simulink library "Contact_Forces_Lib"  (R2018a)
settings: Solver=ode45  StartTime=0.0  StopTime=10.0  RelTol=1e-3  EnableMultiTasking=on
undefined symbols (not defined in the file or in its folder): b_contact, custom_param_1, custom_param_2, k_contact, l_cone, length_cylinder, length_tube, mu_kinetic, mu_static, pen_exponent, pen_full_damp_F, rad_s_cone, radius_cylinder, radius_tube, v_thr, X, Y, Z
libraries: nesl_utility x153, sm_lib x64, $bdroot x53, simulink x9, fl_lib x1
(part 6 of 7)

== system Contact_Forces_Lib/3D/Sphere to Tube Force/Sensing/rad_azm_cal ==
  X : Inport
  Y : Inport  Port=2
  Xdot : Inport  Port=3
  Ydot : Inport  Port=4
  Demux : Demux
  If centers are not colocated : If  IfExpression=(u1 > 0)
  Math Function : Math  Operator=square  SaturateOnIntegerOverflow=on
  Math Function1 : Math  Operator=square  SaturateOnIntegerOverflow=on
  Merge : Merge  InitialOutput=0  InputPortOffsets=0
  Sum : Sum  Inputs=|++
  rad_0 : Subsystem
  rad_azm_cal : Subsystem
  rad : Outport
  azm : Outport  Port=2
  radv : Outport  Port=3
  azmv : Outport  Port=4
  wires:
  Merge/1 -> Demux/1
  If centers are not colocated/1 -> rad_azm_cal/Action
  If centers are not colocated/2 -> rad_0/Action
  Demux/2 -> azm/1
  rad_0/1(F) -> Merge/1
  Demux/4 -> azmv/1
  Demux/1 -> rad/1
  Demux/3 -> radv/1
  Xdot/1 -> rad_azm_cal/3(Xdot)
  X/1 -> Math Function/1, rad_azm_cal/1(X)
  Ydot/1 -> rad_azm_cal/4(Ydot)
  Y/1 -> Math Function1/1, rad_azm_cal/2(Y)
  rad_azm_cal/1(F) -> Merge/2
  Math Function1/1 -> Sum/2
  Math Function/1 -> Sum/1
  Sum/1 -> If centers are not colocated/1

== system Contact_Forces_Lib/Friction Utilities/Utilities/Product/FcConst ==
  PS Product : fl_lib/Physical Signals/Functions/PS Product
      settings: SourceProductName=Simscape
  PS-Simulink Converter2 : nesl_utility/PS-Simulink Converter  PhysicalDomain=network_engine_domain  SubClassName=ps_output  LeftPortType=input  RightPortType=output  PseudoPeriodic=off  Frequencies=[]  Unit=1  AffineConversion=off
  Terminator : Terminator
  Fc : PMIOPort  Side=Right
  v : PMIOPort  Port=2  Side=Right
  wires:
  PS-Simulink Converter2/1 -> Terminator/1
  connections:
  PS Product/LConn1 -- v/RConn1
  PS Product/LConn2 -- Fc/RConn1
  PS-Simulink Converter2/LConn1 -- PS Product/RConn1

== system Contact_Forces_Lib/Friction Utilities/Utilities/Product/FcVect ==
  PS-Simulink Converter1 : nesl_utility/PS-Simulink Converter  PhysicalDomain=network_engine_domain  SubClassName=ps_output  LeftPortType=input  RightPortType=output  PseudoPeriodic=off  Frequencies=[]  Unit=1  AffineConversion=off
  PS-Simulink Converter2 : nesl_utility/PS-Simulink Converter  PhysicalDomain=network_engine_domain  SubClassName=ps_output  LeftPortType=input  RightPortType=output  PseudoPeriodic=off  Frequencies=[]  Unit=1  AffineConversion=off
  Terminator : Terminator
  Terminator1 : Terminator
  Fc : PMIOPort  Side=Right
  v : PMIOPort  Port=2  Side=Right
  wires:
  PS-Simulink Converter1/1 -> Terminator1/1
  PS-Simulink Converter2/1 -> Terminator/1
  connections:
  PS-Simulink Converter1/LConn1 -- Fc/RConn1
  PS-Simulink Converter2/LConn1 -- v/RConn1

== system Contact_Forces_Lib/2D/Circle to Circle Force/Ff/Resolve Ff/Ff in CirB ==
  Ff : Inport
  azm : Inport  Port=2
  Divide1 : Product  Inputs=**
  Divide2 : Product  Inputs=**
  Gain3 : Gain  Gain=-1
  cos : Trigonometry
  deg2rad : Gain  Gain=pi/180
  sin : Trigonometry  Operator=cos
  FxCirB : Outport
  FyCirB : Outport  Port=2
  wires:
  Gain3/1 -> Divide1/2
  Ff/1 -> Divide1/1, Divide2/1
  Divide1/1 -> FxCirB/1
  deg2rad/1 -> cos/1, sin/1
  sin/1 -> Divide2/2
  cos/1 -> Gain3/1
  Divide2/1 -> FyCirB/1  "Fy Cir"
  azm/1 -> deg2rad/1

== system Contact_Forces_Lib/2D/Circle to Circle Force/Ff/Resolve Ff/Ff in CirF ==
  R : Inport
  FxCirB : Inport  Port=2
  FyCirB : Inport  Port=3
  Demux : Demux  Outputs=2
  Divide3 : Product  Inputs=**  Multiplication=Matrix(*)
  Gain1 : Gain  Gain=-1
  Mux1 : Mux  Inputs=2
  FyCirF : Outport
  FxCirF : Outport  Port=2
  wires:
  FxCirB/1 -> Mux1/2
  FyCirB/1 -> Mux1/1
  Demux/2 -> FxCirF/1
  Demux/1 -> FyCirF/1
  Gain1/1 -> Demux/1
  Mux1/1 -> Divide3/2
  Divide3/1 -> Gain1/1
  R/1 -> Divide3/1

== system Contact_Forces_Lib/2D/Circle to Circle Force/Ff/Resolve Ff/Tz ==
  Ff : Inport
  Base Radius : Constant  Value=cirB_rad
  Divide4 : Product  Inputs=**
  Divide5 : Product  Inputs=**
  Follower Radius : Constant  Value=cirF_rad
  Gain2 : Gain
  TzB : Outport
  TzF : Outport  Port=2
  wires:
  Ff/1 -> Divide4/2, Gain2/1
  Gain2/1 -> Divide5/1
  Divide4/1 -> TzF/1
  Follower Radius/1 -> Divide4/1
  Divide5/1 -> TzB/1
  Base Radius/1 -> Divide5/2

== system Contact_Forces_Lib/2D/Circle to Circle Force Enabled/Ff/Resolve Ff/Ff in CirB ==
  Ff : Inport
  azm : Inport  Port=2
  Divide1 : Product  Inputs=**
  Divide2 : Product  Inputs=**
  Gain3 : Gain  Gain=-1
  cos : Trigonometry
  deg2rad : Gain  Gain=pi/180
  sin : Trigonometry  Operator=cos
  FxCirB : Outport
  FyCirB : Outport  Port=2
  wires:
  azm/1 -> deg2rad/1
  Divide2/1 -> FyCirB/1  "Fy Cir"
  cos/1 -> Gain3/1
  sin/1 -> Divide2/2
  deg2rad/1 -> sin/1, cos/1
  Divide1/1 -> FxCirB/1
  Ff/1 -> Divide2/1, Divide1/1
  Gain3/1 -> Divide1/2

== system Contact_Forces_Lib/2D/Circle to Circle Force Enabled/Ff/Resolve Ff/Ff in CirF ==
  R : Inport
  FxCirB : Inport  Port=2
  FyCirB : Inport  Port=3
  Demux : Demux  Outputs=2
  Divide3 : Product  Inputs=**  Multiplication=Matrix(*)
  Gain1 : Gain  Gain=-1
  Mux1 : Mux  Inputs=2
  FyCirF : Outport
  FxCirF : Outport  Port=2
  wires:
  R/1 -> Divide3/1
  Divide3/1 -> Gain1/1
  Mux1/1 -> Divide3/2
  Gain1/1 -> Demux/1
  Demux/1 -> FyCirF/1
  Demux/2 -> FxCirF/1
  FyCirB/1 -> Mux1/1
  FxCirB/1 -> Mux1/2

== system Contact_Forces_Lib/2D/Circle to Circle Force Enabled/Ff/Resolve Ff/Tz ==
  Ff : Inport
  Base Radius : Constant  Value=cirB_rad
  Divide4 : Product  Inputs=**
  Divide5 : Product  Inputs=**
  Follower Radius : Constant  Value=cirF_rad
  Gain2 : Gain
  TzB : Outport
  TzF : Outport  Port=2
  wires:
  Base Radius/1 -> Divide5/2
  Divide5/1 -> TzB/1
  Follower Radius/1 -> Divide4/1
  Divide4/1 -> TzF/1
  Gain2/1 -> Divide5/1
  Ff/1 -> Gain2/1, Divide4/2

== system Contact_Forces_Lib/2D/Circle to Finite Line Force/Forces/Resolve Forces/FnCir ==
  note: Calculate circle Normal Force in circle reference frame
  Unit Vector : Inport
  Fn : Inport  Port=2
  Demux1 : Demux  Outputs=2
  Divide1 : Product  Inputs=**
  FxCir : Outport
  FyCir : Outport  Port=2
  wires:
  Unit Vector/1 -> Divide1/2
  Divide1/1 -> Demux1/1
  Fn/1 -> Divide1/1
  Demux1/2 -> FyCir/1  "Fy Cir"
  Demux1/1 -> FxCir/1  "Fx Cir"

== system Contact_Forces_Lib/2D/Circle to Finite Line Force/Forces/Resolve Forces/FnLin ==
  note: Normal Force is calculated in line reference frame,
      | and acts along x-axis only.
  Fn : Inport
  Constant : Constant  Value=0
  Constant1 : Constant  Value=0
  Sum : Sum
  FxLin : Outport
  FyLin : Outport  Port=2
  wires:
  Constant1/1 -> Sum/1
  Sum/1 -> FxLin/1
  Fn/1 -> Sum/2  "Fx Lin"
  Constant/1 -> FyLin/1  "Fy Lin"

== system Contact_Forces_Lib/2D/Circle to Finite Line Force/Forces/Resolve Forces/Friction ==
  Unit Vector : Inport
  Fn : Inport  Port=2
  X Sep : Inport  Port=3
  vLin : Inport  Port=4
  wz : Inport  Port=5
  Components : Gain  Gain=[1 -1]
  Demux : Demux  Outputs=2
  Friction Law : $bdroot/Friction Law  OverrideUsingVariant=None
  Line Ref h : Gain  Gain=line_depth
  Product1 : Product
  Product2 : Product
  Product3 : Product
  Radius : Gain  Gain=-circle_rad
  Sign : Signum
  Sum : Sum  Inputs=-+
  VCirPt : Subsystem
  FxCir : Outport
  FyCir : Outport  Port=2
  FyLin : Outport  Port=3
  TzLin : Outport  Port=4
  TzCir : Outport  Port=5
  Ff : Outport  Port=6
  wires:
  Sign/1 -> Product3/2, Product1/2
  X Sep/1 -> VCirPt/2(X sep), Sign/1
  Product2/1 -> Demux/1
  Radius/1 -> TzCir/1
  Line Ref h/1 -> TzLin/1
  Fn/1 -> Friction Law/1
  Sum/1 -> Friction Law/2
  Unit Vector/1 -> Components/1
  wz/1 -> VCirPt/1(wz)
  Demux/2 -> FxCir/1  "FxCir"
  VCirPt/1(vCir) -> Sum/2
  vLin/1 -> Sum/1
  Demux/1 -> FyCir/1  "FyCir"
  Friction Law/1 -> Product1/1, Radius/1, Ff/1, Product2/2, Line Ref h/1  "Ff"
  Product1/1 -> FyLin/1
  Components/1 -> Product3/1
  Product3/1 -> Product2/1

== system Contact_Forces_Lib/2D/Circle to Finite Line Force Enabled/Forces/Resolve Forces/FnCir ==
  note: Calculate circle Normal Force in circle reference frame
  Unit Vector : Inport
  Fn : Inport  Port=2
  Demux1 : Demux  Outputs=2
  Divide1 : Product  Inputs=**
  FxCir : Outport
  FyCir : Outport  Port=2
  wires:
  Demux1/1 -> FxCir/1  "Fx Cir"
  Demux1/2 -> FyCir/1  "Fy Cir"
  Fn/1 -> Divide1/1
  Divide1/1 -> Demux1/1
  Unit Vector/1 -> Divide1/2

== system Contact_Forces_Lib/2D/Circle to Finite Line Force Enabled/Forces/Resolve Forces/FnLin ==
  note: Normal Force is calculated in line reference frame,
      | and acts along x-axis only.
  Fn : Inport
  Constant : Constant  Value=0
  Constant1 : Constant  Value=0
  Sum : Sum
  FxLin : Outport
  FyLin : Outport  Port=2
  wires:
  Constant/1 -> FyLin/1  "Fy Lin"
  Fn/1 -> Sum/2  "Fx Lin"
  Sum/1 -> FxLin/1
  Constant1/1 -> Sum/1

== system Contact_Forces_Lib/2D/Circle to Finite Line Force Enabled/Forces/Resolve Forces/Friction ==
  Unit Vector : Inport
  Fn : Inport  Port=2
  X Sep : Inport  Port=3
  vLin : Inport  Port=4
  wz : Inport  Port=5
  Components : Gain  Gain=[1 -1]
  Demux : Demux  Outputs=2
  Friction Law : $bdroot/Friction Law  OverrideUsingVariant=None
  Line Ref h : Gain  Gain=line_depth
  Product1 : Product
  Product2 : Product
  Product3 : Product
  Radius : Gain  Gain=-circle_rad
  Sign : Signum
  Sum : Sum  Inputs=-+
  VCirPt : Subsystem
  FxCir : Outport
  FyCir : Outport  Port=2
  FyLin : Outport  Port=3
  TzLin : Outport  Port=4
  TzCir : Outport  Port=5
  Ff : Outport  Port=6
  wires:
  Product3/1 -> Product2/1
  Components/1 -> Product3/1
  Product1/1 -> FyLin/1
  Friction Law/1 -> Line Ref h/1, Product2/2, Ff/1, Radius/1, Product1/1  "Ff"
  Demux/1 -> FyCir/1  "FyCir"
  vLin/1 -> Sum/1
  VCirPt/1(vCir) -> Sum/2
  Demux/2 -> FxCir/1  "FxCir"
  wz/1 -> VCirPt/1(wz)
  Unit Vector/1 -> Components/1
  Sum/1 -> Friction Law/2
  Fn/1 -> Friction Law/1
  Line Ref h/1 -> TzLin/1
  Radius/1 -> TzCir/1
  Product2/1 -> Demux/1
  X Sep/1 -> Sign/1, VCirPt/2(X sep)
  Sign/1 -> Product1/2, Product3/2

== system Contact_Forces_Lib/2D/Circle to Ring Force/Forces/Ff/Resolve Ff ==
  note: Resolve Friction Force in
      | Circle B reference frame
      | Sign of Fn indicates
      | inside or outside ring.
  note: Resolve Friction Force in
      | Circle F reference frame
  Fn : Inport
  R : Inport  Port=2
  Ff : Inport  Port=3
  azm : Inport  Port=4
  Ff in CirB : Subsystem
  Ff in CirF : Subsystem
  Product : Product
  Sign : Signum  ZeroCross=off
  Tz : Subsystem
  FxCirF : Outport
  FyCirF : Outport  Port=2
  TzCirF : Outport  Port=3
  FxRinB : Outport  Port=4
  FyRinB : Outport  Port=5
  TzRinB : Outport  Port=6
  wires:
  Product/1 -> Ff in CirB/1(Ff)
  Sign/1 -> Product/2
  Fn/1 -> Sign/1
  Ff in CirF/1(FyCirF) -> FyCirF/1
  Ff in CirB/1(FxRinB) -> FxRinB/1, Ff in CirF/2(FxRinB)
  Ff in CirB/2(FyRinB) -> FyRinB/1, Ff in CirF/3(FyRinB)
  Ff in CirF/2(FxCirF) -> FxCirF/1
  Ff/1 -> Product/1, Tz/1(Ff)
  Tz/1(TzRinB) -> TzRinB/1
  Tz/2(TzCirF) -> TzCirF/1
  azm/1 -> Ff in CirB/2(azm)
  R/1 -> Ff in CirF/1(R)

== system Contact_Forces_Lib/2D/Circle to Ring Force/Forces/Ff/vTan ==
  Fn : Inport
  rad : Inport  Port=2
  Pen : Inport  Port=3
  vazm : Inport  Port=4
  wzf : Inport  Port=5
  Follower Radius : Constant  Value=radius_circle
  Midpt Pen : Gain  Gain=0.5
  Product1 : Product
  Product2 : Product
  Product3 : Product  Inputs=3
  Sign : Signum  ZeroCross=off
  Sum : Sum  Inputs=++-
  Sum1 : Sum  Inputs=+-
  Sum2 : Sum  Inputs=-+
  vTan : Outport
  wires:
  Sign/1 -> Product1/2, Product3/3
  Fn/1 -> Sign/1
  Product1/1 -> Sum/3
  Sum2/1 -> vTan/1
  Pen/1 -> Midpt Pen/1
  Sum/1 -> Product2/2
  rad/1 -> Sum/2
  Product2/1 -> Sum2/2  "vTan in B"
  Product3/1 -> Sum2/1  "vTan of F"
  Follower Radius/1 -> Sum1/1, Product1/1
  wzf/1 -> Product3/1
  vazm/1 -> Product2/1
  Midpt Pen/1 -> Sum1/2, Sum/1
  Sum1/1 -> Product3/2

== system Contact_Forces_Lib/2D/Circle to Ring Force/Forces/Fn/Fn in CirB ==
  Fn : Inport
  azm : Inport  Port=2
  Divide1 : Product  Inputs=**
  Divide2 : Product  Inputs=**
  Gain2 : Gain  Gain=-1
  cos : Trigonometry  Operator=cos
  deg2rad : Gain  Gain=pi/180
  sin : Trigonometry
  FxCirB : Outport
  FyCirB : Outport  Port=2
  wires:
  Gain2/1 -> Divide1/1, Divide2/1
  deg2rad/1 -> cos/1, sin/1
  sin/1 -> Divide2/2
  cos/1 -> Divide1/2
  Divide1/1 -> FxCirB/1
  Divide2/1 -> FyCirB/1
  Fn/1 -> Gain2/1
  azm/1 -> deg2rad/1

== system Contact_Forces_Lib/2D/Circle to Ring Force/Forces/Fn/Fn in CirF ==
  R : Inport
  FxCirB : Inport  Port=2
  FyCirB : Inport  Port=3
  Demux : Demux  Outputs=2
  Divide3 : Product  Inputs=**  Multiplication=Matrix(*)
  Gain : Gain  Gain=-1
  Mux1 : Mux  Inputs=2
  FyCirF : Outport
  FxCirF : Outport  Port=2
  wires:
  Demux/2 -> FxCirF/1
  Demux/1 -> FyCirF/1
  Gain/1 -> Demux/1
  Mux1/1 -> Divide3/2
  Divide3/1 -> Gain/1
  R/1 -> Divide3/1
  FyCirB/1 -> Mux1/1
  FxCirB/1 -> Mux1/2

== system Contact_Forces_Lib/2D/Composite Forces/Box to Belt Force/Belt Ends/Sensing C5 ==
  S : Inport
  Bus Selector : BusSelector  OutputSignals=Normal Force
  Fn : Outport
  wires:
  S/1 -> Bus Selector/1
  Bus Selector/1 -> Fn/1  "<Normal Force>"

== system Contact_Forces_Lib/2D/Composite Forces/Box to Belt Force/Belt Ends/Sensing C6 ==
  S : Inport
  Bus Selector : BusSelector  OutputSignals=Normal Force
  Fn : Outport
  wires:
  Bus Selector/1 -> Fn/1  "<Normal Force>"
  S/1 -> Bus Selector/1

== system Contact_Forces_Lib/2D/Composite Forces/Box to Belt Force/Belt Ends/Sensing C7 ==
  S : Inport
  Bus Selector : BusSelector  OutputSignals=Normal Force
  Fn : Outport
  wires:
  Bus Selector/1 -> Fn/1  "<Normal Force>"
  S/1 -> Bus Selector/1

== system Contact_Forces_Lib/2D/Composite Forces/Box to Belt Force/Belt Ends/Sensing C8 ==
  S : Inport
  Bus Selector : BusSelector  OutputSignals=Normal Force
  Fn : Outport
  wires:
  S/1 -> Bus Selector/1
  Bus Selector/1 -> Fn/1  "<Normal Force>"

== system Contact_Forces_Lib/2D/Composite Forces/Box to Belt Force/Belt Faces/Sensing C1 ==
  S : Inport
  Bus Selector : BusSelector  OutputSignals=Normal Force
  Fn : Outport
  wires:
  Bus Selector/1 -> Fn/1  "<Normal Force>"
  S/1 -> Bus Selector/1

== system Contact_Forces_Lib/2D/Composite Forces/Box to Belt Force/Belt Faces/Sensing C2 ==
  S : Inport
  Bus Selector : BusSelector  OutputSignals=Normal Force
  Fn : Outport
  wires:
  S/1 -> Bus Selector/1
  Bus Selector/1 -> Fn/1  "<Normal Force>"

== system Contact_Forces_Lib/2D/Composite Forces/Box to Belt Force/Belt Faces/Sensing C3 ==
  S : Inport
  Bus Selector : BusSelector  OutputSignals=Normal Force
  Fn : Outport
  wires:
  S/1 -> Bus Selector/1
  Bus Selector/1 -> Fn/1  "<Normal Force>"

== system Contact_Forces_Lib/2D/Composite Forces/Box to Belt Force/Belt Faces/Sensing C4 ==
  S : Inport
  Bus Selector : BusSelector  OutputSignals=Normal Force
  Fn : Outport
  wires:
  Bus Selector/1 -> Fn/1  "<Normal Force>"
  S/1 -> Bus Selector/1

== system Contact_Forces_Lib/2D/Composite Forces/Box to Box Force/BoxB Corners/Forces ==
  1AC : Inport
  1BD : Inport  Port=2
  2AC : Inport  Port=3
  2BD : Inport  Port=4
  3AC : Inport  Port=5
  3BD : Inport  Port=6
  4AC : Inport  Port=7
  4BD : Inport  Port=8
  Bus Creator : BusCreator  Inputs=8
  Bus Selector{1..8} (8 alike) : BusSelector  OutputSignals=FLin.Fx  OutputAsBus=on
  tag scope: FrcBC=scoped
  wires:
  Bus Creator/1 -> [FrcBC]
  Bus Selector7/1 -> Bus Creator/8  "BC4BD"
  4BD/1 -> Bus Selector7/1
  Bus Selector8/1 -> Bus Creator/7  "BC4AC"
  4AC/1 -> Bus Selector8/1
  Bus Selector5/1 -> Bus Creator/6  "BC3BD"
  3BD/1 -> Bus Selector5/1
  Bus Selector6/1 -> Bus Creator/5  "BC3AC"
  3AC/1 -> Bus Selector6/1
  Bus Selector3/1 -> Bus Creator/4  "BC2BD"
  2BD/1 -> Bus Selector3/1
  Bus Selector4/1 -> Bus Creator/3  "BC2AC"
  2AC/1 -> Bus Selector4/1
  Bus Selector1/1 -> Bus Creator/2  "BC1BD"
  1BD/1 -> Bus Selector1/1
  Bus Selector2/1 -> Bus Creator/1  "BC1AC"
  1AC/1 -> Bus Selector2/1

== system Contact_Forces_Lib/2D/Composite Forces/Box to Box Force/BoxF Corners/Forces ==
  1AC : Inport
  1BD : Inport  Port=2
  2AC : Inport  Port=3
  2BD : Inport  Port=4
  3AC : Inport  Port=5
  3BD : Inport  Port=6
  4AC : Inport  Port=7
  4BD : Inport  Port=8
  Bus Creator : BusCreator  Inputs=8
  Bus Selector{1..8} (8 alike) : BusSelector  OutputSignals=FLin.Fx  OutputAsBus=on
  tag scope: FrcFC=scoped
  wires:
  Bus Creator/1 -> [FrcFC]
  Bus Selector7/1 -> Bus Creator/8  "FC4BD"
  4BD/1 -> Bus Selector7/1
  Bus Selector8/1 -> Bus Creator/7  "FC4AC"
  4AC/1 -> Bus Selector8/1
  Bus Selector5/1 -> Bus Creator/6  "FC3BD"
  3BD/1 -> Bus Selector5/1
  Bus Selector6/1 -> Bus Creator/5  "FC3AC"
  3AC/1 -> Bus Selector6/1
  Bus Selector3/1 -> Bus Creator/4  "FC2BD"
  2BD/1 -> Bus Selector3/1
  Bus Selector4/1 -> Bus Creator/3  "FC2AC"
  2AC/1 -> Bus Selector4/1
  Bus Selector1/1 -> Bus Creator/2  "FC1BD"
  1BD/1 -> Bus Selector1/1
  Bus Selector2/1 -> Bus Creator/1  "FC1AC"
  1AC/1 -> Bus Selector2/1

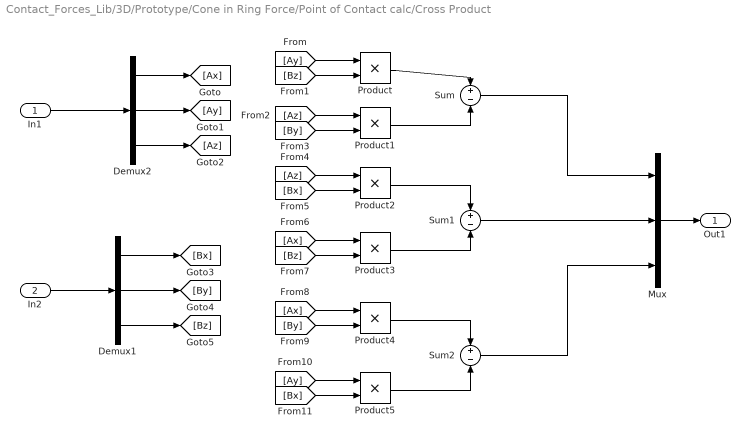
== system Contact_Forces_Lib/3D/Prototype/Cone in Ring Force/Point of Contact calc/Cross Product ==
  In1 : Inport
  In2 : Inport  Port=2
  Demux1 : Demux  Outputs=3
  Demux2 : Demux  Outputs=3
  Mux : Mux  Inputs=3
  Product{,1..5} (6 alike) : Product
  Sum : Sum  Inputs=+|-
  Sum1 : Sum  Inputs=+|-
  Sum2 : Sum  Inputs=+|-
  Out1 : Outport
  wires:
  [Bx] -> Product5/2
  [Ay] -> Product5/1
  [By] -> Product4/2
  [Ax] -> Product4/1
  [Bz] -> Product3/2
  [Ax] -> Product3/1
  [Bx] -> Product2/2
  [Az] -> Product2/1
  [By] -> Product1/2
  [Az] -> Product1/1
  [Bz] -> Product/2
  [Ay] -> Product/1
  Demux1/3 -> [Bz]
  Demux1/2 -> [By]
  Demux1/1 -> [Bx]
  Demux2/3 -> [Az]
  Demux2/2 -> [Ay]
  Demux2/1 -> [Ax]
  In1/1 -> Demux2/1
  Sum2/1 -> Mux/3
  Sum/1 -> Mux/1
  Sum1/1 -> Mux/2
  Product5/1 -> Sum2/2
  Product4/1 -> Sum2/1
  Product3/1 -> Sum1/2
  Product2/1 -> Sum1/1
  Product/1 -> Sum/1
  Product1/1 -> Sum/2
  Mux/1 -> Out1/1
  In2/1 -> Demux1/1

== system Contact_Forces_Lib/3D/Prototype/Cone in Ring Force/Point of Contact calc/Force Calc ==
  x : Inport
  y : Inport  Port=2
  r : Inport  Port=3
  z : Inport  Port=4
  th : Inport  Port=5
  Computing Force from nonzero penetration points : Subsystem  Commented=on
  Constant2 : Constant  Value=r_tube
  Dead Zone : DeadZone  LowerValue=-inf  UpperValue=0  ZeroCross=off  SaturateOnIntegerOverflow=on
  MAX_ML : Subsystem  Commented=on
  MAX_SL : Subsystem
  Math Function : Math  Operator=square  SaturateOnIntegerOverflow=on
  Math Function1 : Math  Operator=square  SaturateOnIntegerOverflow=on
  Reciprocal Sqrt : Sqrt  SaturateOnIntegerOverflow=on
  Sum : Sum  Inputs=|++
  Sum1 : Sum  Inputs=|+-
  Fx : Outport
  Fy : Outport  Port=2
  Fz : Outport  Port=3
  pc : Outport  Port=4
  wires:
  x/1 -> MAX_SL/2(X), Math Function/1
  Sum/1 -> Reciprocal Sqrt/1
  Reciprocal Sqrt/1 -> Sum1/1
  Constant2/1 -> Sum1/2
  Sum1/1 -> Dead Zone/1
  Math Function1/1 -> Sum/1
  Math Function/1 -> Sum/2
  y/1 -> Math Function1/1, MAX_SL/1(Y)
  MAX_SL/1(Fx) -> Fx/1
  MAX_SL/2(Fy) -> Fy/1
  Dead Zone/1 -> MAX_SL/3(Pen)
  MAX_SL/3(Fz) -> Fz/1
  MAX_SL/4(pc) -> pc/1
  r/1 -> MAX_SL/4(r)
  th/1 -> MAX_SL/5(th)
  z/1 -> MAX_SL/6(z)

== system Contact_Forces_Lib/3D/Prototype/Cone in Ring Force/Point of Contact calc/r calc ==
  note: r(z) = (z+l_cyl/2)(rl-rs)/lc +rl
  z : Inport
  Constant4 : Constant  Value=(rl + (l_cyl*(rl - rs))/(2*lc))
  Gain1 : Gain  Gain=(rl - rs)/lc
  Sum1 : Sum  Inputs=|++
  r : Outport
  wires:
  Constant4/1 -> Sum1/2
  Gain1/1 -> Sum1/1
  z/1 -> Gain1/1
  Sum1/1 -> r/1

== system Contact_Forces_Lib/3D/Prototype/Cone in Ring Force/Point of Contact calc/x calc ==
  r11 : Inport
  r12 : Inport  Port=2
  r13 : Inport  Port=3
  xc : Inport  Port=4
  th : Inport  Port=5
  z : Inport  Port=6
  r : Inport  Port=7
  Product{,1..4} (5 alike) : Product
  Sum : Sum  Inputs=|++++
  Trigonometric Function : Trigonometry  Operator=cos
  Trigonometric Function1 : Trigonometry
  x : Outport
  wires:
  th/1 -> Trigonometric Function1/1, Trigonometric Function/1
  Sum/1 -> x/1
  Product/1 -> Product3/1
  Product4/1 -> Sum/3
  Trigonometric Function/1 -> Product/2
  Trigonometric Function1/1 -> Product1/2
  Product3/1 -> Sum/2
  Product1/1 -> Product4/2
  r11/1 -> Product/1
  r12/1 -> Product1/1
  xc/1 -> Sum/1
  r13/1 -> Product2/1
  z/1 -> Product2/2
  Product2/1 -> Sum/4
  r/1 -> Product3/2, Product4/1

== system Contact_Forces_Lib/3D/Prototype/Cone in Ring Force/Point of Contact calc/y calc ==
  r21 : Inport
  r22 : Inport  Port=2
  r23 : Inport  Port=3
  yc : Inport  Port=4
  th : Inport  Port=5
  z : Inport  Port=6
  r : Inport  Port=7
  Product{,1..4} (5 alike) : Product
  Sum : Sum  Inputs=|++++
  Trigonometric Function : Trigonometry  Operator=cos
  Trigonometric Function1 : Trigonometry
  y : Outport
  wires:
  Product2/1 -> Sum/4
  z/1 -> Product2/2
  r23/1 -> Product2/1
  yc/1 -> Sum/1
  r22/1 -> Product1/1
  r21/1 -> Product/1
  Product1/1 -> Product4/2
  Product3/1 -> Sum/2
  Trigonometric Function1/1 -> Product1/2
  Trigonometric Function/1 -> Product/2
  Product4/1 -> Sum/3
  Product/1 -> Product3/1
  Sum/1 -> y/1
  th/1 -> Trigonometric Function1/1, Trigonometric Function/1
  r/1 -> Product3/2, Product4/1

== system Contact_Forces_Lib/3D/Prototype/Cone in Ring Force/Point of Contact calc/z calc ==
  note: num = -(Zc - L/2 + r31*cos(th)*(rl + (Lcyl*(rl - rs))/(2*lc)) + r32*sin(th)*(rl + (Lcyl*(rl - rs))/(2*lc)))
      | den = (r33 + (r31*cos(th)*(rl - rs))/lc + (r32*sin(th)*(rl - rs))/lc)
  r31 : Inport
  r32 : Inport  Port=2
  r33 : Inport  Port=3
  zc : Inport  Port=4
  th : Inport  Port=5
  Constant : Constant  Value=(rl + (l_cyl*(rl - rs))/(2*lc))
  Constant1 : Constant  Value=l_tube/2
  Constant2 : Constant  Value=(rl - rs)/lc
  Divide : Product  Inputs=*/
  Gain : Gain  Gain=-1
  Product{,1..5} (6 alike) : Product
  Sum : Sum  Inputs=+-++
  Sum1 : Sum  Inputs=+++
  Trigonometric Function : Trigonometry  Operator=cos
  Trigonometric Function1 : Trigonometry
  z : Outport
  wires:
  Divide/1 -> z/1
  th/1 -> Trigonometric Function1/1, Trigonometric Function/1
  Trigonometric Function/1 -> Product/2
  r31/1 -> Product/1
  Trigonometric Function1/1 -> Product1/2
  r32/1 -> Product1/1
  zc/1 -> Sum/1
  Constant1/1 -> Sum/2
  Product2/1 -> Sum/3
  Product3/1 -> Sum/4
  Product/1 -> Product4/1, Product2/1
  Product1/1 -> Product3/1, Product5/1
  Constant/1 -> Product3/2, Product2/2
  Sum/1 -> Gain/1
  Product5/1 -> Sum1/3
  Product4/1 -> Sum1/2
  r33/1 -> Sum1/1
  Constant2/1 -> Product4/2, Product5/2
  Sum1/1 -> Divide/2
  Gain/1 -> Divide/1

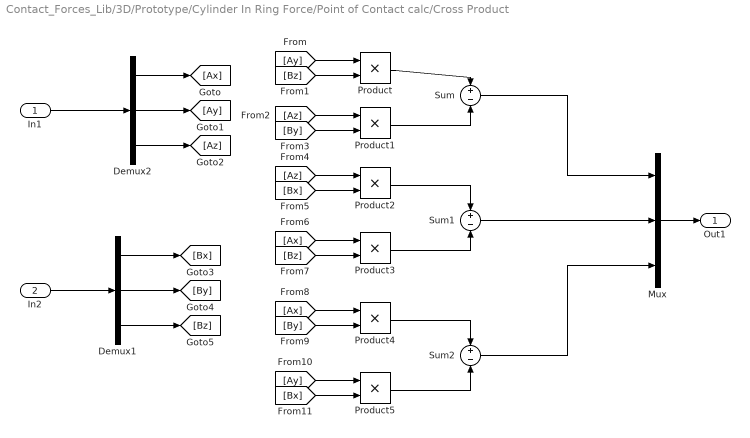
== system Contact_Forces_Lib/3D/Prototype/Cylinder In Ring Force/Point of Contact calc/Cross Product ==
  In1 : Inport
  In2 : Inport  Port=2
  Demux1 : Demux  Outputs=3
  Demux2 : Demux  Outputs=3
  Mux : Mux  Inputs=3
  Product{,1..5} (6 alike) : Product
  Sum : Sum  Inputs=+|-
  Sum1 : Sum  Inputs=+|-
  Sum2 : Sum  Inputs=+|-
  Out1 : Outport
  wires:
  [Bx] -> Product5/2
  [Ay] -> Product5/1
  [By] -> Product4/2
  [Ax] -> Product4/1
  [Bz] -> Product3/2
  [Ax] -> Product3/1
  [Bx] -> Product2/2
  [Az] -> Product2/1
  [By] -> Product1/2
  [Az] -> Product1/1
  [Bz] -> Product/2
  [Ay] -> Product/1
  Demux1/3 -> [Bz]
  Demux1/2 -> [By]
  Demux1/1 -> [Bx]
  Demux2/3 -> [Az]
  Demux2/2 -> [Ay]
  Demux2/1 -> [Ax]
  In1/1 -> Demux2/1
  Sum2/1 -> Mux/3
  Sum/1 -> Mux/1
  Sum1/1 -> Mux/2
  Product5/1 -> Sum2/2
  Product4/1 -> Sum2/1
  Product3/1 -> Sum1/2
  Product2/1 -> Sum1/1
  Product/1 -> Sum/1
  Product1/1 -> Sum/2
  Mux/1 -> Out1/1
  In2/1 -> Demux1/1

== system Contact_Forces_Lib/3D/Prototype/Cylinder In Ring Force/Point of Contact calc/Force Calc ==
  x : Inport
  y : Inport  Port=2
  v : Inport  Port=3
  z : Inport  Port=4
  th : Inport  Port=5
  Computing Force from nonzero penetration points : Subsystem  Commented=on
  Constant2 : Constant  Value=r_tube
  Dead Zone : DeadZone  LowerValue=-inf  UpperValue=0  ZeroCross=off  SaturateOnIntegerOverflow=on
  MAX_ML : Subsystem  Commented=on
  MAX_SL : Subsystem
  Math Function : Math  Operator=square  SaturateOnIntegerOverflow=on
  Math Function1 : Math  Operator=square  SaturateOnIntegerOverflow=on
  Reciprocal Sqrt : Sqrt  SaturateOnIntegerOverflow=on
  Sum : Sum  Inputs=|++
  Sum1 : Sum  Inputs=|+-
  Fx : Outport
  Fy : Outport  Port=2
  Fz : Outport  Port=3
  pc : Outport  Port=4
  maxpen : Outport  Port=5
  wires:
  y/1 -> MAX_SL/1(Y), Math Function1/1
  x/1 -> MAX_SL/2(X), Math Function/1
  Sum/1 -> Reciprocal Sqrt/1
  Reciprocal Sqrt/1 -> Sum1/1
  Constant2/1 -> Sum1/2
  Sum1/1 -> Dead Zone/1
  MAX_SL/1(Fx) -> Fx/1
  MAX_SL/2(Fy) -> Fy/1
  Dead Zone/1 -> MAX_SL/3(Pen)
  Math Function1/1 -> Sum/1
  Math Function/1 -> Sum/2
  v/1 -> MAX_SL/4(v)
  th/1 -> MAX_SL/5(th)
  z/1 -> MAX_SL/6(z)
  MAX_SL/4(pc) -> pc/1
  MAX_SL/3(Fz) -> Fz/1
  MAX_SL/5(maxpen) -> maxpen/1

== system Contact_Forces_Lib/3D/Prototype/Cylinder In Ring Force/Point of Contact calc/x calc ==
  note: Xb = r11*r*cos(th) + r12*r*sin(th) +r13*z + Xc;
  note: Find x coordinate in tube frame for cylinder point that is in the plane of the end of the tube
  r11 : Inport
  r12 : Inport  Port=2
  r13 : Inport  Port=3
  xc : Inport  Port=4
  th : Inport  Port=5
  z : Inport  Port=6
  Gain : Gain  Gain=r_cyl
  Gain1 : Gain  Gain=r_cyl
  Product : Product
  Product1 : Product
  Product2 : Product
  Sum : Sum  Inputs=|++++
  Trigonometric Function : Trigonometry  Operator=cos
  Trigonometric Function1 : Trigonometry
  x : Outport
  wires:
  th/1 -> Trigonometric Function/1, Trigonometric Function1/1
  Sum/1 -> x/1
  Product/1 -> Gain/1
  Gain1/1 -> Sum/3
  Trigonometric Function/1 -> Product/2
  Trigonometric Function1/1 -> Product1/2
  Gain/1 -> Sum/2
  Product1/1 -> Gain1/1
  r11/1 -> Product/1
  r12/1 -> Product1/1
  xc/1 -> Sum/1
  r13/1 -> Product2/1
  z/1 -> Product2/2
  Product2/1 -> Sum/4

== system Contact_Forces_Lib/3D/Prototype/Cylinder In Ring Force/Point of Contact calc/y calc ==
  note: Yb = r21*r*cos(th) + r22*r*sin(th) +r23*z + Yc;
  note: Find y coordinate in tube frame for cylinder point that is in the plane of the end of the tube
  r21 : Inport
  r22 : Inport  Port=2
  r23 : Inport  Port=3
  yc : Inport  Port=4
  th : Inport  Port=5
  z : Inport  Port=6
  Gain : Gain  Gain=r_cyl
  Gain1 : Gain  Gain=r_cyl
  Product : Product
  Product1 : Product
  Product2 : Product
  Sum : Sum  Inputs=|++++
  Trigonometric Function : Trigonometry  Operator=cos
  Trigonometric Function1 : Trigonometry
  y : Outport
  wires:
  Product2/1 -> Sum/4
  z/1 -> Product2/2
  r23/1 -> Product2/1
  yc/1 -> Sum/1
  r22/1 -> Product1/1
  r21/1 -> Product/1
  Product1/1 -> Gain1/1
  Gain/1 -> Sum/2
  Trigonometric Function1/1 -> Product1/2
  Trigonometric Function/1 -> Product/2
  Gain1/1 -> Sum/3
  Product/1 -> Gain/1
  Sum/1 -> y/1
  th/1 -> Trigonometric Function1/1, Trigonometric Function/1

== system Contact_Forces_Lib/3D/Prototype/Cylinder In Ring Force/Point of Contact calc/z calc ==
  note: Find z coordinate in cylinder frame for cylinder point that is in the plane of the end of the tube
  note: z = (L/2 - r31*r*cos(th) - r32*r*sin(th) - Zc)/r33;
  r31 : Inport
  r32 : Inport  Port=2
  r33 : Inport  Port=3
  zc : Inport  Port=4
  th : Inport  Port=5
  Constant : Constant  Value=l_tube/2
  Divide : Product  Inputs=*/
  Gain : Gain  Gain=r_cyl
  Gain1 : Gain  Gain=r_cyl
  Product : Product
  Product1 : Product
  Sum : Sum  Inputs=|---+
  Trigonometric Function : Trigonometry  Operator=cos
  Trigonometric Function1 : Trigonometry
  z : Outport
  wires:
  r32/1 -> Product1/1
  r31/1 -> Product/1
  Product1/1 -> Gain1/1
  Gain/1 -> Sum/2
  Trigonometric Function1/1 -> Product1/2
  Trigonometric Function/1 -> Product/2
  Gain1/1 -> Sum/3
  Product/1 -> Gain/1
  r33/1 -> Divide/2
  Constant/1 -> Sum/4
  Sum/1 -> Divide/1
  Divide/1 -> z/1
  zc/1 -> Sum/1
  th/1 -> Trigonometric Function1/1, Trigonometric Function/1

== system Contact_Forces_Lib/3D/Sphere in Sphere Force/Ff/Check w or v non zero/Else ==
  Action Port : ActionPort
  vabs_zero : Constant  Value=0  SampleTime=0
  vuvect_zero : Constant  Value=[0 0 0]  SampleTime=0
  vabs : Outport  InitialOutput=0
  vuvect : Outport  Port=2  InitialOutput=0
  wires:
  vabs_zero/1 -> vabs/1
  vuvect_zero/1 -> vuvect/1

== system Contact_Forces_Lib/3D/Sphere in Sphere Force/Ff/Check w or v non zero/mag v ==
  vect : Inport
  Add2 : Sum  Inputs=+++
  Demux : Demux  Outputs=3
  Math Function : Math  Operator=square  SaturateOnIntegerOverflow=on
  Math Function1 : Math  Operator=square  SaturateOnIntegerOverflow=on
  Math Function2 : Math  Operator=square  SaturateOnIntegerOverflow=on
  Sqrt : Sqrt  SaturateOnIntegerOverflow=on
  mag : Outport
  wires:
  Math Function2/1 -> Add2/3
  Demux/3 -> Math Function2/1
  Sqrt/1 -> mag/1
  Math Function1/1 -> Add2/2
  Math Function/1 -> Add2/1
  Add2/1 -> Sqrt/1
  vect/1 -> Demux/1
  Demux/1 -> Math Function/1
  Demux/2 -> Math Function1/1

== system Contact_Forces_Lib/3D/Sphere in Sphere Force/Ff/Check w or v non zero/mag w ==
  vect : Inport
  Add : Sum  Inputs=+++
  Demux : Demux  Outputs=3
  Math Function : Math  Operator=square  SaturateOnIntegerOverflow=on
  Math Function1 : Math  Operator=square  SaturateOnIntegerOverflow=on
  Math Function2 : Math  Operator=square  SaturateOnIntegerOverflow=on
  Sqrt : Sqrt  SaturateOnIntegerOverflow=on
  mag : Outport
  wires:
  Demux/2 -> Math Function1/1
  Demux/1 -> Math Function/1
  vect/1 -> Demux/1
  Add/1 -> Sqrt/1
  Math Function/1 -> Add/1
  Math Function1/1 -> Add/2
  Sqrt/1 -> mag/1
  Demux/3 -> Math Function2/1
  Math Function2/1 -> Add/3

== system Contact_Forces_Lib/3D/Sphere in Sphere Force/Ff/SlipVel/If Action Subsystem ==
  In1 : Inport
  In2 : Inport  Port=2
  Action Port : ActionPort
  Divide : Product  Inputs=/*
  Out1 : Outport
  wires:
  Divide/1 -> Out1/1
  In2/1 -> Divide/2
  In1/1 -> Divide/1

== system Contact_Forces_Lib/3D/Sphere in Sphere Force/Ff/SlipVel/mag ==
  vect : Inport
  Add2 : Sum  Inputs=+++
  Demux : Demux  Outputs=3
  Math Function : Math  Operator=square  SaturateOnIntegerOverflow=on
  Math Function1 : Math  Operator=square  SaturateOnIntegerOverflow=on
  Math Function2 : Math  Operator=square  SaturateOnIntegerOverflow=on
  Sqrt : Sqrt  SaturateOnIntegerOverflow=on
  mag : Outport
  wires:
  Math Function2/1 -> Add2/3
  Demux/3 -> Math Function2/1
  Sqrt/1 -> mag/1
  Math Function1/1 -> Add2/2
  Math Function/1 -> Add2/1
  Add2/1 -> Sqrt/1
  vect/1 -> Demux/1
  Demux/1 -> Math Function/1
  Demux/2 -> Math Function1/1

== system Contact_Forces_Lib/3D/Sphere to Plane Force/Forces/Ff/SlipVel ==
  wx : Inport
  wy : Inport  Port=2
  vx : Inport  Port=3
  vy : Inport  Port=4
  Fx1 : Constant  Value=sphere_rad
  Math Function : Math  Operator=square  SaturateOnIntegerOverflow=on
  Math Function1 : Math  Operator=square  SaturateOnIntegerOverflow=on
  Product3 : Product
  Product4 : Product
  Sqrt : Sqrt  SaturateOnIntegerOverflow=on
  Sum1 : Sum  Inputs=|++
  Sum2 : Sum  Inputs=|-+
  Sum3 : Sum  Inputs=|++
  Trigonometric Function : Trigonometry  Operator=atan2
  vabs : Outport
  alpha : Outport  Port=2
  wires:
  Sum2/1 -> Math Function1/1, Trigonometric Function/2  "slipx"
  Sum1/1 -> Math Function/1, Trigonometric Function/1  "slipy"
  Math Function1/1 -> Sum3/2
  Math Function/1 -> Sum3/1
  Sum3/1 -> Sqrt/1
  Sqrt/1 -> vabs/1
  Trigonometric Function/1 -> alpha/1
  Product4/1 -> Sum2/1
  vy/1 -> Sum1/2
  Fx1/1 -> Product4/1, Product3/2
  vx/1 -> Sum2/2
  wy/1 -> Product4/2
  Product3/1 -> Sum1/1
  wx/1 -> Product3/1

== system Contact_Forces_Lib/3D/Sphere to Sphere Force/Ff/Check w or v non zero/Else ==
  Action Port : ActionPort
  Constant : Constant  Value=0  SampleTime=0
  Constant1 : Constant  Value=[0 0 0]  SampleTime=0
  vabs : Outport  InitialOutput=0
  vuvect : Outport  Port=2  InitialOutput=0
  wires:
  Constant1/1 -> vuvect/1
  Constant/1 -> vabs/1

== system Contact_Forces_Lib/3D/Sphere to Sphere Force/Ff/Check w or v non zero/mag v ==
  vect : Inport
  Add2 : Sum  Inputs=+++
  Demux : Demux  Outputs=3
  Math Function : Math  Operator=square  SaturateOnIntegerOverflow=on
  Math Function1 : Math  Operator=square  SaturateOnIntegerOverflow=on
  Math Function2 : Math  Operator=square  SaturateOnIntegerOverflow=on
  Sqrt : Sqrt  SaturateOnIntegerOverflow=on
  mag : Outport
  wires:
  Demux/2 -> Math Function1/1
  Demux/1 -> Math Function/1
  vect/1 -> Demux/1
  Add2/1 -> Sqrt/1
  Math Function/1 -> Add2/1
  Math Function1/1 -> Add2/2
  Sqrt/1 -> mag/1
  Demux/3 -> Math Function2/1
  Math Function2/1 -> Add2/3

== system Contact_Forces_Lib/3D/Sphere to Sphere Force/Ff/Check w or v non zero/mag w ==
  vect : Inport
  Add : Sum  Inputs=+++
  Demux : Demux  Outputs=3
  Math Function : Math  Operator=square  SaturateOnIntegerOverflow=on
  Math Function1 : Math  Operator=square  SaturateOnIntegerOverflow=on
  Math Function2 : Math  Operator=square  SaturateOnIntegerOverflow=on
  Sqrt : Sqrt  SaturateOnIntegerOverflow=on
  mag : Outport
  wires:
  Math Function2/1 -> Add/3
  Demux/3 -> Math Function2/1
  Sqrt/1 -> mag/1
  Math Function1/1 -> Add/2
  Math Function/1 -> Add/1
  Add/1 -> Sqrt/1
  vect/1 -> Demux/1
  Demux/1 -> Math Function/1
  Demux/2 -> Math Function1/1

== system Contact_Forces_Lib/3D/Sphere to Sphere Force/Ff/SlipVel/If Action Subsystem ==
  In1 : Inport
  In2 : Inport  Port=2
  Action Port : ActionPort
  Divide : Product  Inputs=/*
  Out1 : Outport
  wires:
  In1/1 -> Divide/1
  In2/1 -> Divide/2
  Divide/1 -> Out1/1

== system Contact_Forces_Lib/3D/Sphere to Sphere Force/Ff/SlipVel/mag ==
  vect : Inport
  Add2 : Sum  Inputs=+++
  Demux : Demux  Outputs=3
  Math Function : Math  Operator=square  SaturateOnIntegerOverflow=on
  Math Function1 : Math  Operator=square  SaturateOnIntegerOverflow=on
  Math Function2 : Math  Operator=square  SaturateOnIntegerOverflow=on
  Sqrt : Sqrt  SaturateOnIntegerOverflow=on
  mag : Outport
  wires:
  Demux/2 -> Math Function1/1
  Demux/1 -> Math Function/1
  vect/1 -> Demux/1
  Add2/1 -> Sqrt/1
  Math Function/1 -> Add2/1
  Math Function1/1 -> Add2/2
  Sqrt/1 -> mag/1
  Demux/3 -> Math Function2/1
  Math Function2/1 -> Add2/3

== system Contact_Forces_Lib/3D/Sphere to Tube Force/Forces/Ff/Resolve Ff ==
  note: Resolve Friction Force in
      | Circle F reference frame
  note: Resolve Friction Force in
      | Circle B reference frame
      | Sign of Fn indicates
      | inside or outside ring.
  Fn : Inport
  R : Inport  Port=2
  Ff : Inport  Port=3
  azm : Inport  Port=4
  alpha : Inport  Port=5
  Ff in CirB : Subsystem
  Ff in CirF : Subsystem
  Product : Product
  Sign : Signum  ZeroCross=off
  FxSphF : Outport
  FySphF : Outport  Port=2
  FzSphF : Outport  Port=3
  TSphF : Outport  Port=4
  FxSphB : Outport  Port=5
  FyTubB : Outport  Port=6
  FzTubB : Outport  Port=7
  TTubB : Outport  Port=8
  wires:
  Ff in CirF/4(TSphF) -> TSphF/1
  Ff in CirB/4(TSphF_B) -> Ff in CirF/5(TSphF_B)
  Ff in CirB/5(TTubB) -> TTubB/1
  alpha/1 -> Ff in CirB/3(alpha)
  Ff in CirB/3(FzTubB) -> Ff in CirF/4(FzTubB), FzTubB/1
  Ff in CirF/3(FzSphF) -> FzSphF/1
  R/1 -> Ff in CirF/1(R)
  azm/1 -> Ff in CirB/2(azm)
  Ff/1 -> Product/1
  Ff in CirF/2(FxSphF) -> FxSphF/1
  Ff in CirB/2(FyTubB) -> FyTubB/1, Ff in CirF/3(FyTubB)
  Ff in CirB/1(FxTubB) -> Ff in CirF/2(FxTubB), FxSphB/1
  Ff in CirF/1(FySphF) -> FySphF/1
  Fn/1 -> Sign/1
  Sign/1 -> Product/2, Ff in CirB/4(Sign)
  Product/1 -> Ff in CirB/1(Ff)

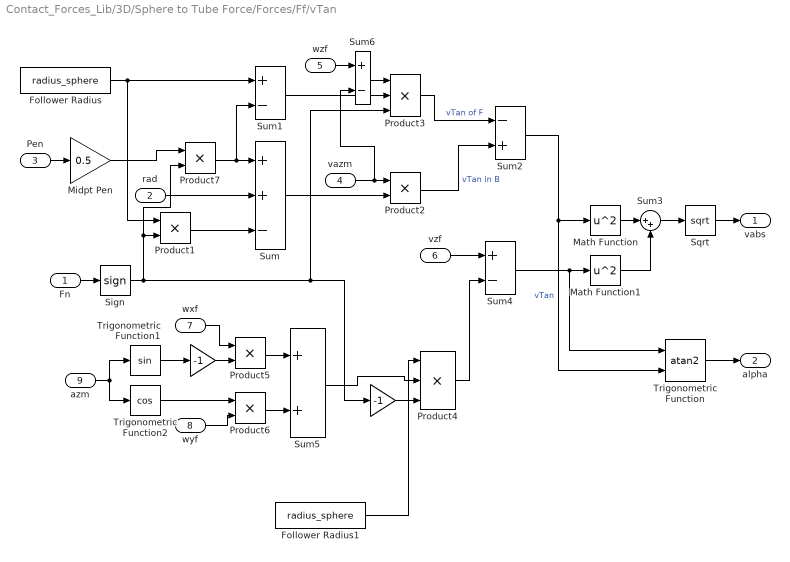
== system Contact_Forces_Lib/3D/Sphere to Tube Force/Forces/Ff/vTan ==
  Fn : Inport
  rad : Inport  Port=2
  Pen : Inport  Port=3
  vazm : Inport  Port=4
  wzf : Inport  Port=5
  vzf : Inport  Port=6
  wxf : Inport  Port=7
  wyf : Inport  Port=8
  azm : Inport  Port=9
  " " : Gain  Gain=-1
  " " : Gain  Gain=-1
  Follower Radius : Constant  Value=radius_sphere
  Follower Radius1 : Constant  Value=radius_sphere
  Math Function : Math  Operator=square  SaturateOnIntegerOverflow=on
  Math Function1 : Math  Operator=square  SaturateOnIntegerOverflow=on
  Midpt Pen : Gain  Gain=0.5
  Product{1..2,5..7} (5 alike) : Product
  Product3 : Product  Inputs=3
  Product4 : Product  Inputs=3
  Sign : Signum  ZeroCross=off
  Sqrt : Sqrt  SaturateOnIntegerOverflow=on
  Sum : Sum  Inputs=++-
  Sum1 : Sum  Inputs=+-
  Sum2 : Sum  Inputs=-+
  Sum3 : Sum  Inputs=|++
  Sum4 : Sum  Inputs=+-
  Sum5 : Sum
  Sum6 : Sum  Inputs=+-
  Trigonometric Function : Trigonometry  Operator=atan2
  Trigonometric Function1 : Trigonometry
  Trigonometric Function2 : Trigonometry  Operator=cos
  vabs : Outport
  alpha : Outport  Port=2
  wires:
  " "/1 -> Product4/3
  Trigonometric Function/1 -> alpha/1
  Sqrt/1 -> vabs/1
  Sum3/1 -> Sqrt/1
  Sum2/1 -> Math Function/1, Trigonometric Function/2  "vTan"
  Math Function/1 -> Sum3/1
  Math Function1/1 -> Sum3/2
  Sum1/1 -> Product3/2
  Product7/1 -> Sum/1, Sum1/2
  vazm/1 -> Sum6/2, Product2/1
  Follower Radius/1 -> Product1/1, Sum1/1
  Product3/1 -> Sum2/1  "vTan of F"
  Product2/1 -> Sum2/2  "vTan in B"
  rad/1 -> Sum/2
  Sum/1 -> Product2/2
  Pen/1 -> Midpt Pen/1
  Product1/1 -> Sum/3
  Fn/1 -> Sign/1
  Sign/1 -> Product3/3, " "/1, Product7/2, Product1/2
  vzf/1 -> Sum4/1
  Product4/1 -> Sum4/2
  Sum4/1 -> Trigonometric Function/1, Math Function1/1
  Trigonometric Function1/1 -> " "/1
  Sum5/1 -> Product4/2
  Product5/1 -> Sum5/1
  wxf/1 -> Product5/1
  " "/1 -> Product5/2
  Product6/1 -> Sum5/2
  Trigonometric Function2/1 -> Product6/1
  wyf/1 -> Product6/2
  azm/1 -> Trigonometric Function1/1, Trigonometric Function2/1
  Follower Radius1/1 -> Product4/1
  Midpt Pen/1 -> Product7/1
  wzf/1 -> Sum6/1
  Sum6/1 -> Product3/1

== system Contact_Forces_Lib/3D/Sphere to Tube Force/Forces/Fn/Fn in SphF ==
  R : Inport
  FxTubB : Inport  Port=2
  FyTubB : Inport  Port=3
  Constant : Constant  Value=0
  Demux : Demux  Outputs=3
  Divide3 : Product  Inputs=/*  Multiplication=Matrix(*)
  Gain : Gain  Gain=-1
  Mux1 : Mux  Inputs=3
  FySphF : Outport
  FxSphF : Outport  Port=2
  FzSphF : Outport  Port=3
  wires:
  Gain/1 -> Demux/1
  R/1 -> Divide3/1
  Constant/1 -> Mux1/3
  Demux/1 -> FxSphF/1
  Demux/2 -> FySphF/1
  Demux/3 -> FzSphF/1
  FxTubB/1 -> Mux1/1
  FyTubB/1 -> Mux1/2
  Mux1/1 -> Divide3/2
  Divide3/1 -> Gain/1

== system Contact_Forces_Lib/3D/Sphere to Tube Force/Forces/Fn/Fn in TubB ==
  Fn : Inport
  azm : Inport  Port=2
  Divide1 : Product  Inputs=**
  Divide2 : Product  Inputs=**
  cos : Trigonometry  Operator=cos
  sin : Trigonometry
  FxTubB : Outport
  FyTubB : Outport  Port=2
  wires:
  Fn/1 -> Divide1/1, Divide2/1
  azm/1 -> cos/1, sin/1
  sin/1 -> Divide2/2
  cos/1 -> Divide1/2
  Divide1/1 -> FxTubB/1
  Divide2/1 -> FyTubB/1

== system Contact_Forces_Lib/3D/Sphere to Tube Force/Sensing/rad_azm_cal/rad_0 ==
  Action Port : ActionPort  ActionType=else
  Zeros : Constant  Value=[0 0 0 0]  SampleTime=0
  F : Outport  InitialOutput=[0]
  wires:
  Zeros/1 -> F/1

== system Contact_Forces_Lib/3D/Sphere to Tube Force/Sensing/rad_azm_cal/rad_azm_cal ==
  note: z = sqrt(x2+y2)
      | zdot = 1/z(x*xdot+y*ydot)
      | azm = atan(y/x)
      | azmdot = 1/z2(x*ydot-xdot*y)
  X : Inport
  Y : Inport  Port=2
  Xdot : Inport  Port=3
  Ydot : Inport  Port=4
  Action Port : ActionPort  ActionType=then
  Add : Sum
  Add1 : Sum  Inputs=+-
  Divide : Product  Inputs=*/
  Divide1 : Product  Inputs=*/
  Math Function : Math  Operator=square  SaturateOnIntegerOverflow=on
  Math Function1 : Math  Operator=square  SaturateOnIntegerOverflow=on
  Mux : Mux
  Product{,1..3} (4 alike) : Product
  Sqrt : Sqrt  SaturateOnIntegerOverflow=on
  Sum : Sum  Inputs=|++
  Trigonometric Function : Trigonometry  Operator=atan2
  F : Outport
  wires:
  Math Function1/1 -> Sum/2
  Math Function/1 -> Sum/1
  Sum/1 -> Divide1/2, Sqrt/1
  Trigonometric Function/1 -> Mux/2
  X/1 -> Trigonometric Function/2, Product2/1, Product/1, Math Function/1
  Y/1 -> Trigonometric Function/1, Product3/1, Product1/1, Math Function1/1
  Xdot/1 -> Product3/2, Product/2
  Ydot/1 -> Product2/2, Product1/2
  Product/1 -> Add/1
  Product1/1 -> Add/2
  Add/1 -> Divide/1
  Sqrt/1 -> Mux/1, Divide/2
  Divide/1 -> Mux/3
  Product2/1 -> Add1/1
  Product3/1 -> Add1/2
  Add1/1 -> Divide1/1
  Divide1/1 -> Mux/4
  Mux/1 -> F/1

== system Contact_Forces_Lib/2D/Circle to Finite Line Force/Forces/Resolve Forces/Friction/VCirPt ==
  wz : Inport
  X sep : Inport  Port=2
  Constant : Constant  Value=line_depth
  Product : Product
  Product1 : Product
  Sign1 : Signum
  Subtract : Sum  Inputs=+-
  vCir : Outport
  wires:
  wz/1 -> Product1/1
  Product1/1 -> vCir/1
  Product/1 -> Subtract/2
  Sign1/1 -> Product/1
  X sep/1 -> Subtract/1, Sign1/1
  Constant/1 -> Product/2
  Subtract/1 -> Product1/2

== system Contact_Forces_Lib/2D/Circle to Finite Line Force Enabled/Forces/Resolve Forces/Friction/VCirPt ==
  wz : Inport
  X sep : Inport  Port=2
  Constant : Constant  Value=line_depth
  Product : Product
  Product1 : Product
  Sign1 : Signum
  Subtract : Sum  Inputs=+-
  vCir : Outport
  wires:
  Subtract/1 -> Product1/2
  Constant/1 -> Product/2
  X sep/1 -> Sign1/1, Subtract/1
  Sign1/1 -> Product/1
  Product/1 -> Subtract/2
  Product1/1 -> vCir/1
  wz/1 -> Product1/1

== system Contact_Forces_Lib/2D/Circle to Ring Force/Forces/Ff/Resolve Ff/Ff in CirB ==
  Ff : Inport
  azm : Inport  Port=2
  Divide1 : Product  Inputs=**
  Divide2 : Product  Inputs=**
  Gain1 : Gain
  Gain3 : Gain  Gain=-1
  cos : Trigonometry
  deg2rad : Gain  Gain=pi/180
  sin : Trigonometry  Operator=cos
  FxRinB : Outport
  FyRinB : Outport  Port=2
  wires:
  Gain1/1 -> Divide2/1, Divide1/1
  azm/1 -> deg2rad/1
  Divide2/1 -> FyRinB/1
  cos/1 -> Gain3/1
  sin/1 -> Divide2/2
  deg2rad/1 -> sin/1, cos/1
  Divide1/1 -> FxRinB/1
  Ff/1 -> Gain1/1
  Gain3/1 -> Divide1/2

== system Contact_Forces_Lib/2D/Circle to Ring Force/Forces/Ff/Resolve Ff/Ff in CirF ==
  R : Inport
  FxRinB : Inport  Port=2
  FyRinB : Inport  Port=3
  Demux : Demux  Outputs=2
  Divide3 : Product  Inputs=**  Multiplication=Matrix(*)
  Gain1 : Gain  Gain=-1
  Mux1 : Mux  Inputs=2
  FyCirF : Outport
  FxCirF : Outport  Port=2
  wires:
  R/1 -> Divide3/1
  Divide3/1 -> Gain1/1
  Mux1/1 -> Divide3/2
  Gain1/1 -> Demux/1
  Demux/1 -> FyCirF/1
  Demux/2 -> FxCirF/1
  FyRinB/1 -> Mux1/1
  FxRinB/1 -> Mux1/2

== system Contact_Forces_Lib/2D/Circle to Ring Force/Forces/Ff/Resolve Ff/Tz ==
  Ff : Inport
  Base Radius : Constant  Value=radius_ring
  Divide4 : Product  Inputs=**
  Divide5 : Product  Inputs=**
  Follower Radius : Constant  Value=radius_circle
  Gain2 : Gain  Gain=-1
  TzRinB : Outport
  TzCirF : Outport  Port=2
  wires:
  Base Radius/1 -> Divide5/2
  Divide5/1 -> TzRinB/1
  Follower Radius/1 -> Divide4/1
  Divide4/1 -> TzCirF/1
  Gain2/1 -> Divide5/1
  Ff/1 -> Gain2/1, Divide4/2

== system Contact_Forces_Lib/3D/Prototype/Cone in Ring Force/Point of Contact calc/Force Calc/Computing Force from nonzero penetration points ==
  Y : Inport
  X : Inport  Port=2
  Pen : Inport  Port=3
  Derivative : Derivative  Commented=on  CoefficientInTFapproximation=1e-4
  For Each Subsystem1 : Subsystem  Commented=on  TreatAsAtomicUnit=on
  For Iterator Subsystem : Subsystem  Commented=on  TreatAsAtomicUnit=on
  Gain1 : Gain  Commented=on  Gain=-1
  Linear1 : Subsystem  Commented=on  VariantControl=Linear  mask(Linear Force Law){k_pen=1e4, b_penvel=1e3}
      mask prompts: k_pen "Contact Stiffness"; b_penvel "Contact Damping"
      mask help: Implements a contact force law as a linear spring damper. The damping force is applied only as the penetration depth increases.
      mask Help: web(which('Force_Laws.html'));
  Product2 : Product  Commented=on
  Product3 : Product  Commented=on
  Sum of Elements : Sum  Commented=on  Inputs=+
  Sum of Elements1 : Sum  Commented=on  Inputs=+
  Sum3 : Sum  Commented=on  Inputs=|+-
  Trigonometric Function3 : Trigonometry  Commented=on  Operator=atan2
  Trigonometric Function4 : Trigonometry  Commented=on  Operator=cos
  Trigonometric Function5 : Trigonometry  Commented=on
  Fx : Outport
  Fy : Outport  Port=2
  wires:
  Trigonometric Function3/1 -> Trigonometric Function5/1, Trigonometric Function4/1
  Linear1/2(Damp F) -> Sum3/2
  Trigonometric Function5/1 -> Product3/1
  Trigonometric Function4/1 -> Product2/1
  Gain1/1 -> Product2/2, Product3/2
  Sum3/1 -> Gain1/1
  Linear1/1(Spr F) -> Sum3/1
  Sum of Elements1/1 -> Fy/1
  Pen/1 -> Derivative/1, For Each Subsystem1/1(In1), Linear1/1(Pen)
  X/1 -> Trigonometric Function3/2
  Y/1 -> Trigonometric Function3/1
  Sum of Elements/1 -> Fx/1
  Derivative/1 -> Linear1/2(Pen Vel)
  Product2/1 -> Sum of Elements/1
  Product3/1 -> Sum of Elements1/1

== system Contact_Forces_Lib/3D/Prototype/Cone in Ring Force/Point of Contact calc/Force Calc/MAX_ML ==
  Y : Inport
  X : Inport  Port=2
  pen : Inport  Port=3
  Gain : Gain  Gain=-1
  Linear : Subsystem  VariantControl=Linear  mask(Linear Force Law){k_pen=k_stiff, b_penvel=b_damp}
      mask prompts: k_pen "Contact Stiffness"; b_penvel "Contact Damping"
      mask help: Implements a contact force law as a linear spring damper. The damping force is applied only as the penetration depth increases.
      mask Help: web(which('Force_Laws.html'));
  MATLAB Function : MATLAB Function  TreatAsAtomicUnit=on
  Product : Product
  Product1 : Product
  Sum2 : Sum  Inputs=|+-
  Transfer Fcn : TransferFcn  Numerator=[1 0]  Denominator=[1e-4 1]
  Trigonometric Function : Trigonometry  Operator=atan2
  Trigonometric Function1 : Trigonometry  Operator=cos
  Trigonometric Function2 : Trigonometry
  Fx : Outport
  Fy : Outport  Port=2
  wires:
  Product1/1 -> Fy/1
  MATLAB Function/4(ind) -> ?
  X/1 -> MATLAB Function/2(x)
  Product/1 -> Fx/1
  pen/1 -> MATLAB Function/1(pen)
  Transfer Fcn/1 -> Linear/2(Pen Vel)
  Gain/1 -> Product1/2, Product/2
  Trigonometric Function1/1 -> Product/1
  Linear/1(Spr F) -> Sum2/1
  Trigonometric Function2/1 -> Product1/1
  Sum2/1 -> Gain/1
  Linear/2(Damp F) -> Sum2/2
  Trigonometric Function/1 -> Trigonometric Function1/1, Trigonometric Function2/1
  Y/1 -> MATLAB Function/3(y)
  MATLAB Function/2(yc) -> Trigonometric Function/1
  MATLAB Function/1(xc) -> Trigonometric Function/2
  MATLAB Function/3(penc) -> Transfer Fcn/1, Linear/1(Pen)

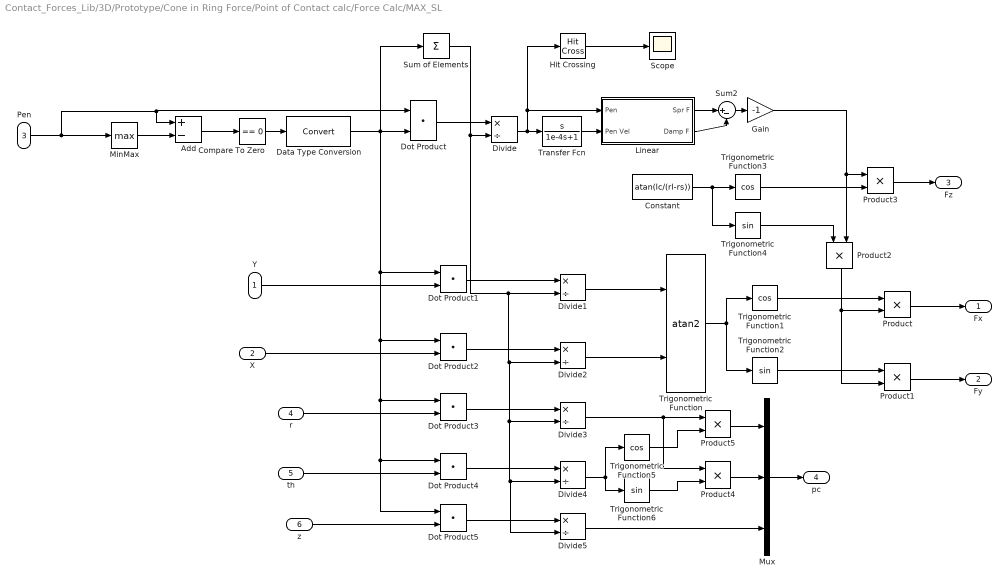
== system Contact_Forces_Lib/3D/Prototype/Cone in Ring Force/Point of Contact calc/Force Calc/MAX_SL ==
  Y : Inport
  X : Inport  Port=2
  Pen : Inport  Port=3
  r : Inport  Port=4
  th : Inport  Port=5
  z : Inport  Port=6
  Add : Sum  Inputs=+-
  Compare To Zero : simulink/Logic and Bit Operations/Compare To Zero  relop===  OutDataTypeStr=boolean  ZeroCross=off
  Constant : Constant  Value=atan(lc/(rl-rs))
  Data Type Conversion : DataTypeConversion
  Divide{,1..5} (6 alike) : Product  Inputs=*/
  Dot Product{,1..5} (6 alike) : DotProduct  InputSameDT=on  OutDataTypeStr=Inherit: Inherit via internal rule
  Gain : Gain  Gain=-1
  Hit Crossing : HitCross
  Linear : Subsystem  VariantControl=Linear  mask(Linear Force Law){k_pen=k_stiff, b_penvel=b_damp}
      mask prompts: k_pen "Contact Stiffness"; b_penvel "Contact Damping"
      mask help: Implements a contact force law as a linear spring damper. The damping force is applied only as the penetration depth increases.
      mask Help: web(which('Force_Laws.html'));
  MinMax : MinMax  Function=max  ZeroCross=off
  Mux : Mux  Inputs=3
  Product{,1..5} (6 alike) : Product
  Scope : Scope
  Sum of Elements : Sum  Inputs=+
  Sum2 : Sum  Inputs=|+-
  Transfer Fcn : TransferFcn  Numerator=[1 0]  Denominator=[1e-4 1]
  Trigonometric Function : Trigonometry  Operator=atan2
  Trigonometric Function1 : Trigonometry  Operator=cos
  Trigonometric Function2 : Trigonometry
  Trigonometric Function3 : Trigonometry  Operator=cos
  Trigonometric Function4 : Trigonometry
  Trigonometric Function5 : Trigonometry  Operator=cos
  Trigonometric Function6 : Trigonometry
  Fx : Outport
  Fy : Outport  Port=2
  Fz : Outport  Port=3
  pc : Outport  Port=4
  wires:
  Trigonometric Function/1 -> Trigonometric Function2/1, Trigonometric Function1/1
  Linear/2(Damp F) -> Sum2/2
  Sum2/1 -> Gain/1
  Trigonometric Function2/1 -> Product1/1
  Linear/1(Spr F) -> Sum2/1
  Trigonometric Function1/1 -> Product/1
  Transfer Fcn/1 -> Linear/2(Pen Vel)
  MinMax/1 -> Add/2
  Add/1 -> Compare To Zero/1
  Compare To Zero/1 -> Data Type Conversion/1
  Product/1 -> Fx/1
  Pen/1 -> Dot Product/1, Add/1, MinMax/1
  Product1/1 -> Fy/1
  Y/1 -> Dot Product1/2
  X/1 -> Dot Product2/2
  Data Type Conversion/1 -> Dot Product/2, Dot Product1/1, Dot Product5/1, Dot Product4/1, Dot Product3/1, Dot Product2/1, Sum of Elements/1
  Dot Product/1 -> Divide/1
  Sum of Elements/1 -> Divide1/2, Divide5/2, Divide4/2, Divide3/2, Divide2/2, Divide/2
  Dot Product1/1 -> Divide1/1
  Dot Product2/1 -> Divide2/1
  Divide1/1 -> Trigonometric Function/1
  Divide2/1 -> Trigonometric Function/2
  Divide/1 -> Hit Crossing/1, Linear/1(Pen), Transfer Fcn/1
  Hit Crossing/1 -> Scope/1
  Constant/1 -> Trigonometric Function4/1, Trigonometric Function3/1
  Trigonometric Function4/1 -> Product2/1
  Gain/1 -> Product3/1, Product2/2
  Product2/1 -> Product1/2, Product/2
  Product3/1 -> Fz/1
  Trigonometric Function3/1 -> Product3/2
  Mux/1 -> pc/1
  Dot Product3/1 -> Divide3/1
  Dot Product4/1 -> Divide4/1
  Dot Product5/1 -> Divide5/1
  r/1 -> Dot Product3/2
  th/1 -> Dot Product4/2
  z/1 -> Dot Product5/2
  Divide5/1 -> Mux/3
  Product4/1 -> Mux/2
  Product5/1 -> Mux/1
  Divide4/1 -> Trigonometric Function5/1, Trigonometric Function6/1
  Divide3/1 -> Product4/1, Product5/1
  Trigonometric Function5/1 -> Product5/2
  Trigonometric Function6/1 -> Product4/2
